simulink model "CA - NonLinear - Simulink"  (R2022b)
settings: Solver=VariableStepAuto  StartTime=0.0  StopTime=500  RelTol=1e-3
undefined symbols (not defined in the file): Gb, Ib, Kd, Kp, n, P1, P2, P3, V
libraries: simulink x2
settings Model: Creator=SHAHAB  LastModifiedBy=SHAHAB

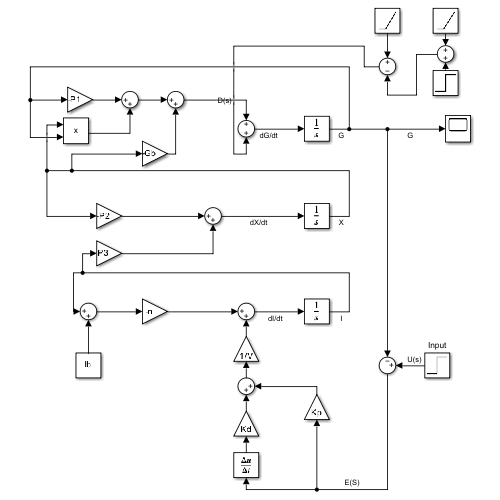
[thumbnail: Simulink's stored preview of the top-level diagram]
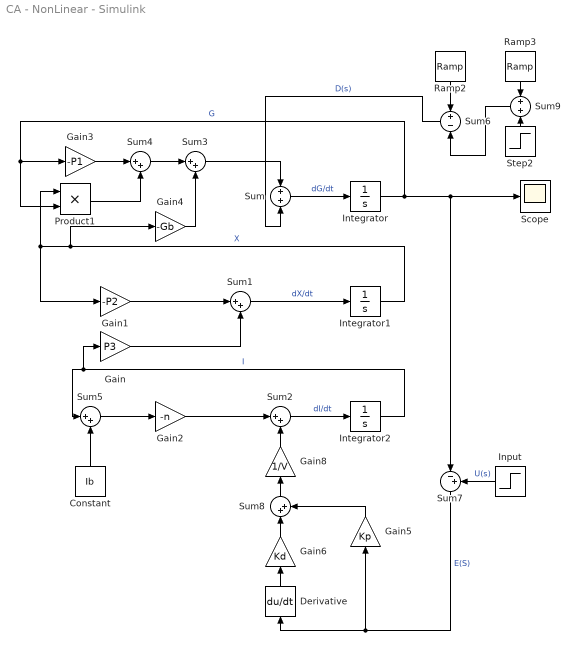
== system CA - NonLinear - Simulink ==
  Constant : Constant  Value=Ib
  Derivative : Derivative
  Gain : Gain  Gain=P3
  Gain1 : Gain  Gain=-P2
  Gain2 : Gain  Gain=-n
  Gain3 : Gain  Gain=-P1
  Gain4 : Gain  Gain=-Gb
  Gain5 : Gain  Gain=Kp
  Gain6 : Gain  Gain=Kd
  Gain8 : Gain  Gain=1/V
  Input : Step  SampleTime=0
  Integrator : Integrator
  Integrator1 : Integrator
  Integrator2 : Integrator
  Product1 : Product
  Ramp2 : simulink/Sources/Ramp  slope=0.5  start=0  InitialOutput=0
  Ramp3 : simulink/Sources/Ramp  slope=0.5  start=1  InitialOutput=0
  Scope : Scope
  Step2 : Step  After=0.5  SampleTime=1
  Sum : Sum
  Sum{1..5,8} (6 alike) : Sum  Inputs=|++
  Sum6 : Sum  Inputs=+-
  Sum7 : Sum  Inputs=|-+
  Sum9 : Sum
  wires:
  Integrator/1 -> Sum7/1, Scope/1, Product1/2, Gain3/1  "G"
  Gain3/1 -> Sum4/1
  Product1/1 -> Sum4/2
  Gain4/1 -> Sum3/2
  Sum4/1 -> Sum3/1
  Integrator1/1 -> Gain1/1, Product1/1, Gain4/1  "X"
  Gain1/1 -> Sum1/1
  Gain/1 -> Sum1/2
  Sum1/1 -> Integrator1/1  "dX/dt"
  Integrator2/1 -> Sum5/1, Gain/1  "I"
  Constant/1 -> Sum5/2
  Sum5/1 -> Gain2/1
  Gain2/1 -> Sum2/1
  Sum2/1 -> Integrator2/1  "dI/dt"
  Input/1 -> Sum7/2  "U(s)"
  Sum7/1 -> Gain5/1, Derivative/1  "E(S)"
  Gain5/1 -> Sum8/2
  Gain8/1 -> Sum2/2
  Sum8/1 -> Gain8/1
  Sum3/1 -> Sum/1
  Sum/1 -> Integrator/1  "dG/dt"
  Sum6/1 -> Sum/2  "D(s)"
  Gain6/1 -> Sum8/1
  Derivative/1 -> Gain6/1
  Ramp3/1 -> Sum9/1
  Sum9/1 -> Sum6/2
  Step2/1 -> Sum9/2
  Ramp2/1 -> Sum6/1
